simulink model "quanser"  (R2023a)
settings: Solver=VariableStepAuto  StartTime=0.0  StopTime=10.0  RelTol=1e-3
values from neighbouring files (symbols this model uses):
  alfa = (1-sin(fi_rad)) / (1+sin(fi_rad))    [proracun.m]
  T = 1 / (sqrt(alfa) * w_c)    [proracun.m]
  Ts = 0    [proracun.m]
undefined symbols (not defined in the file or in its folder): Model_626, Sensoray
libraries: sldrtlib x2
settings Model: Creator=pavij  LastModifiedBy=pavij

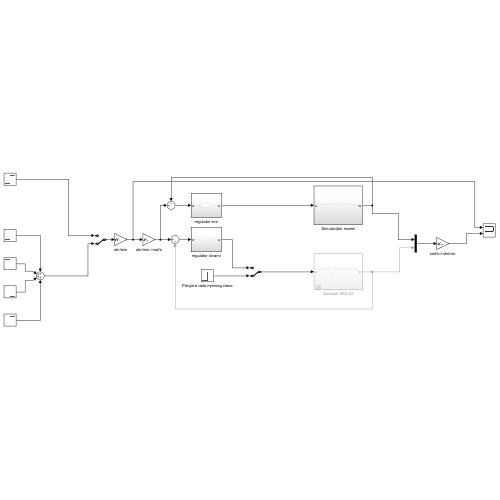
[thumbnail: Simulink's stored preview of the top-level diagram]
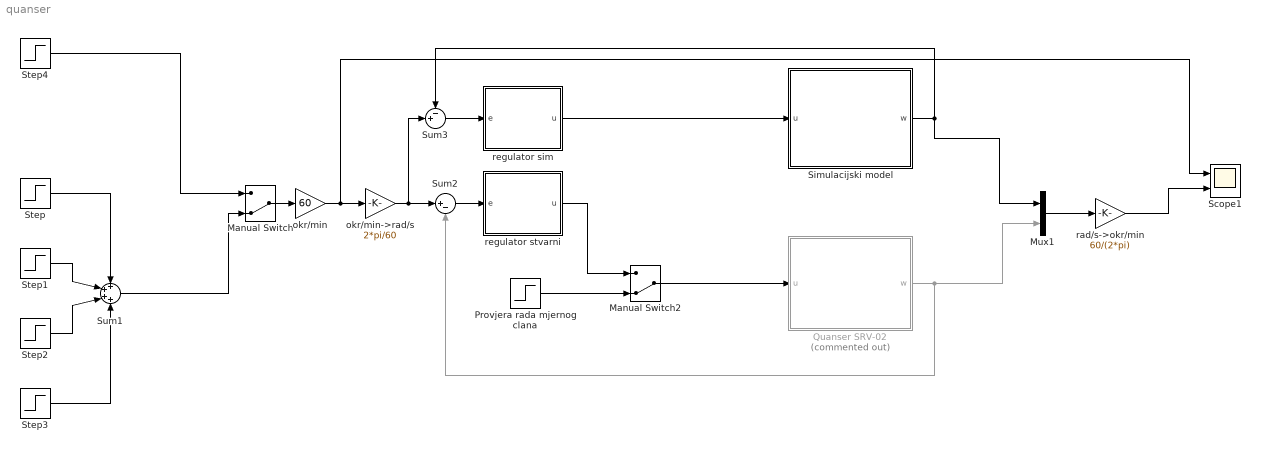
== system quanser ==
  Manual Switch : ManualSwitch  CurrentSetting=0
  Manual Switch2 : ManualSwitch  CurrentSetting=0
  Mux1 : Mux  Inputs=2
  Provjera rada mjernog clana : Step  Time=2  After=3  SampleTime=0
  Quanser SRV-02 : Subsystem  Commented=on
  Scope1 : Scope  NumInputPorts=2
  Simulacijski model : Subsystem
  Step : Step  Time=2  SampleTime=0
  Step1 : Step  Time=4  After=-1  SampleTime=0
  Step2 : Step  Time=6  After=-1  SampleTime=0
  Step3 : Step  Time=8  SampleTime=0
  Step4 : Step  Time=2  SampleTime=0
  Sum1 : Sum  Inputs=++++
  Sum2 : Sum  Inputs=|+-
  Sum3 : Sum  Inputs=-+|
  okr/min : Gain  Gain=60
  okr/min->rad/s : Gain  Gain=2*pi/60
  rad/s->okr/min : Gain  Gain=60/(2*pi)
  regulator sim : Subsystem
  regulator stvarni : Subsystem
  wires:
  Mux1/1 -> rad/s->okr/min/1
  Step1/1 -> Sum1/2
  regulator sim/1(u) -> Simulacijski model/1(u)
  Sum1/1 -> Manual Switch/2
  Step/1 -> Sum1/1
  Provjera rada mjernog clana/1 -> Manual Switch2/2
  rad/s->okr/min/1 -> Scope1/2
  Simulacijski model/1(w) -> Mux1/1, Sum3/1
  Manual Switch/1 -> okr/min/1
  Quanser SRV-02/1(w) -> Mux1/2, Sum2/2
  regulator stvarni/1(u) -> Manual Switch2/1
  Step3/1 -> Sum1/4
  Sum3/1 -> regulator sim/1(e)
  Sum2/1 -> regulator stvarni/1(e)
  Step2/1 -> Sum1/3
  Manual Switch2/1 -> Quanser SRV-02/1(u)
  okr/min/1 -> Scope1/1, okr/min->rad/s/1
  okr/min->rad/s/1 -> Sum3/2, Sum2/1
  Step4/1 -> Manual Switch/1

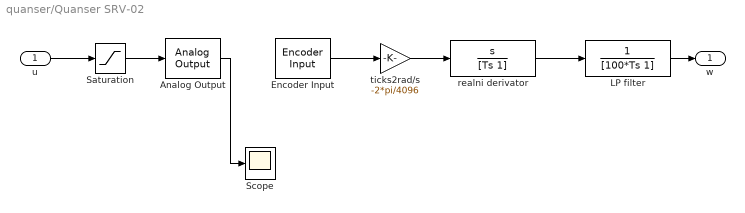
== system quanser/Quanser SRV-02 ==
  u : Inport
  Analog Output : sldrtlib/Analog Output  SampleTime=Ts  MaxMissedTicks=100  ShowMissedTicks=on  YieldWhenWaiting=off  DrvName=Sensoray/Model_626  DrvAddress=4294967295  DrvOptions=zeros(1,0)  Channels=1  RangeMode=1  VoltRange=1  InitialValue=0  FinalValue=0
      settings: AttributesFormatString=Sensoray\nModel 626 [auto]
  Encoder Input : sldrtlib/Encoder Input  SampleTime=Ts  MaxMissedTicks=100  ShowMissedTicks=off  YieldWhenWaiting=off  DrvName=Sensoray/Model_626  DrvAddress=4294967295  DrvOptions=zeros(1,0)  Channels=1  QuadMode=3  IndexPulse=2  InputFilter=Inf  DataType=1
      settings: AttributesFormatString=Sensoray\nModel 626 [auto]
  LP filter : TransferFcn  Denominator=[100*Ts 1]
  Saturation : Saturate  UpperLimit=6  LowerLimit=-6
  Scope : Scope
  realni derivator : TransferFcn  Numerator=[1 0]  Denominator=[Ts 1]
  ticks2rad/s : Gain  Gain=-2*pi/4096
  w : Outport
  wires:
  Encoder Input/1 -> ticks2rad/s/1
  ticks2rad/s/1 -> realni derivator/1
  Analog Output/1 -> Scope/1
  realni derivator/1 -> LP filter/1
  LP filter/1 -> w/1
  u/1 -> Saturation/1
  Saturation/1 -> Analog Output/1

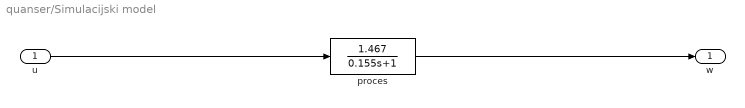
== system quanser/Simulacijski model ==
  u : Inport
  proces : TransferFcn  Numerator=[1.467]  Denominator=[0.155 1]
  w : Outport
  wires:
  proces/1 -> w/1
  u/1 -> proces/1

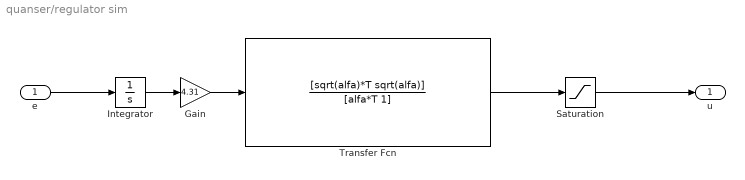
== system quanser/regulator sim ==
  e : Inport
  Gain : Gain  Gain=4.31
  Integrator : Integrator
  Saturation : Saturate  UpperLimit=6  LowerLimit=-6
  Transfer Fcn : TransferFcn  Numerator=[sqrt(alfa)*T sqrt(alfa)]  Denominator=[alfa*T 1]
  u : Outport
  wires:
  e/1 -> Integrator/1
  Saturation/1 -> u/1
  Integrator/1 -> Gain/1
  Transfer Fcn/1 -> Saturation/1
  Gain/1 -> Transfer Fcn/1

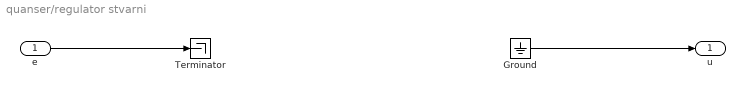
== system quanser/regulator stvarni ==
  e : Inport
  Ground : Ground
  Terminator : Terminator
  u : Outport
  wires:
  e/1 -> Terminator/1
  Ground/1 -> u/1
